simulink model "P2_Q6"  (R2023a)
settings: Solver=VariableStepAuto  StartTime=0.0  StopTime=20  RelTol=1e-3
settings Model: Creator=asus  LastModifiedBy=asus

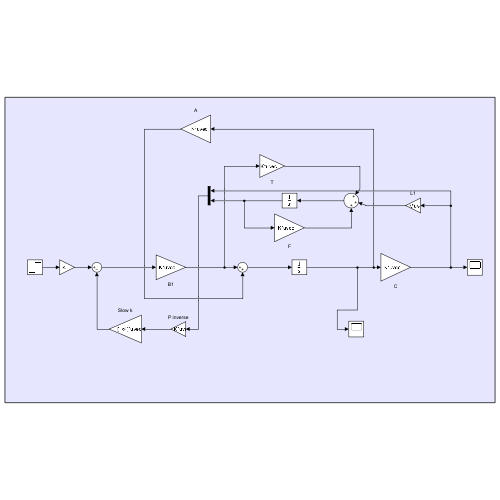
[thumbnail: Simulink's stored preview of the top-level diagram]
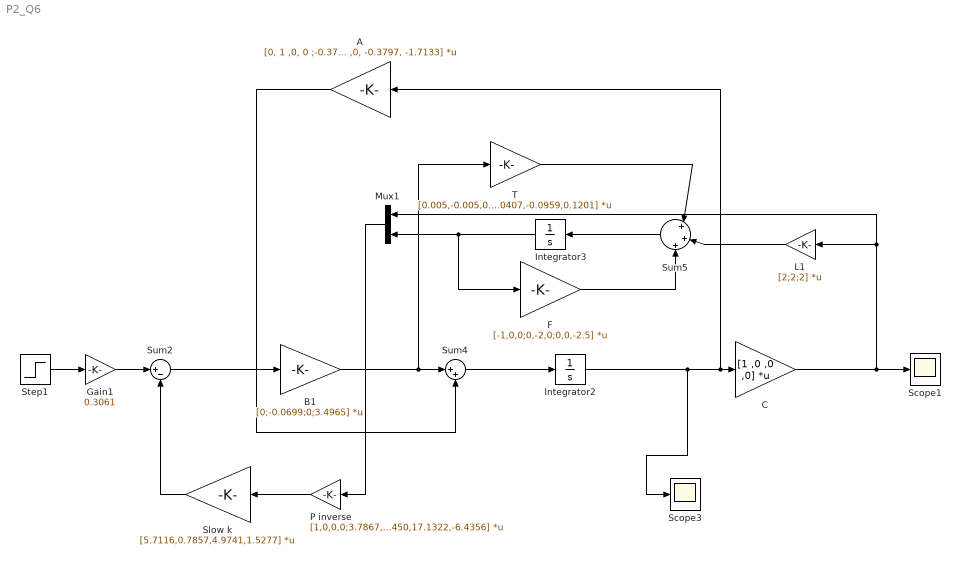
== system P2_Q6 ==
  A : Gain  Gain=[0, 1 ,0, 0 ;-0.378 ,0 ,7.0147 ,0.0343;0, 0, 0, 1; 18.9001 ,0, -0.3797, -1.7133]  Multiplication=Matrix(K*u) (u vector)
  B1 : Gain  Gain=[0;-0.0699;0;3.4965]  Multiplication=Matrix(K*u) (u vector)
  C : Gain  Gain=[1 ,0 ,0 ,0]  Multiplication=Matrix(K*u) (u vector)
  F : Gain  Gain=[-1,0,0;0,-2,0;0,0,-2.5]  Multiplication=Matrix(K*u) (u vector)
  Gain1 : Gain  Gain=0.3061
  Integrator2 : Integrator
  Integrator3 : Integrator
  L1 : Gain  Gain=[2;2;2]  Multiplication=Matrix(K*u) (u vector)
  Mux1 : Mux  Inputs=2
  P inverse : Gain  Gain=[1,0,0,0;3.7867,44.1305,-127.1110,76.9382;0.3760,17.5363,-32.4604,14.1445;-0.1356,-0.9450,17.1322,-6.4356]  Multiplication=Matrix(K*u) (u vector)
  Scope1 : Scope
  Scope3 : Scope
  Slow k : Gain  Gain=[5.7116,0.7857,4.9741,1.5277]  Multiplication=Matrix(K*u) (u vector)
  Step1 : Step  Time=0  After=0.1  SampleTime=0
  Sum2 : Sum  Inputs=|+-
  Sum4 : Sum  Inputs=|++
  Sum5 : Sum  Inputs=|+|+|+
  T : Gain  Gain=[0.005,-0.005,0.0754,0.1055;-0.03,0.0150,-0.0319,0.1093;-0.1017,0.0407,-0.0959,0.1201]  Multiplication=Matrix(K*u) (u vector)
  wires:
  Sum5/1 -> Integrator3/1
  Mux1/1 -> P inverse/1
  T/1 -> Sum5/1
  Step1/1 -> Gain1/1
  Sum2/1 -> B1/1
  Integrator3/1 -> F/1, Mux1/2
  L1/1 -> Sum5/2
  B1/1 -> Sum4/1, T/1
  Gain1/1 -> Sum2/1
  Sum4/1 -> Integrator2/1
  A/1 -> Sum4/2
  C/1 -> L1/1, Mux1/1, Scope1/1
  F/1 -> Sum5/3
  Integrator2/1 -> A/1, C/1, Scope3/1
  P inverse/1 -> Slow k/1
  Slow k/1 -> Sum2/2
